simulink model "work"  (R2023a)
settings: Solver=FixedStepDiscrete  StartTime=1  StopTime=16  FixedStep=1  RelTol=1e-3
model workspace (MAT data in the model file):
  efwed = 0
undefined symbols (not defined in the file or in its folder): kfailsoftroll, mode
libraries: simulink x7
settings Model: DataDictionary=data.sldd  Creator=23208  LastModifiedBy=23208
settings DataIOCC: ExternalInput=[cycle, leftAdverseYaw,rightAdverseYaw,joystickCmd,expectationrollrate,OffPressed,expectationleftwarning,expectationrightwarning,expectationmode]  LoadExternalInput=on

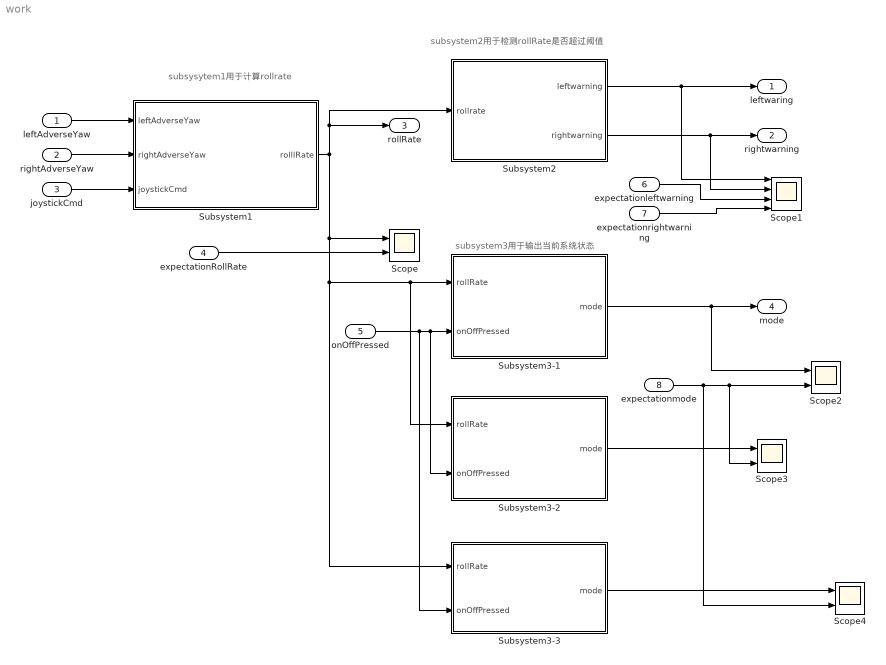
== system work ==
  note: subsystem2用于检测rollRate是否超过阈值
  note: subsysytem1用于计算rollrate
  note: subsystem3用于输出当前系统状态
  leftAdverseYaw : Inport  OutDataTypeStr=double
  rightAdverseYaw : Inport  Port=2  OutDataTypeStr=double
  joystickCmd : Inport  Port=3  OutDataTypeStr=double
  expectationRollRate : Inport  Port=4
  onOffPressed : Inport  Port=5
  expectationleftwarning : Inport  Port=6  OutDataTypeStr=double
  expectationrightwarning : Inport  Port=7  OutDataTypeStr=double
  expectationmode : Inport  Port=8
  Scope{,2..4} (4 alike) : Scope  NumInputPorts=2
  Scope1 : Scope  NumInputPorts=4
  Subsystem1 : Subsystem
  Subsystem2 : Subsystem
  Subsystem3-1 : Subsystem
  Subsystem3-2 : Subsystem
  Subsystem3-3 : Subsystem
  leftwaring : Outport  OutDataTypeStr=boolean
  rightwarning : Outport  Port=2  OutDataTypeStr=boolean
  rollRate : Outport  Port=3
  mode : Outport  Port=4
  wires:
  leftAdverseYaw/1 -> Subsystem1/1(leftAdverseYaw)
  rightAdverseYaw/1 -> Subsystem1/2(rightAdverseYaw)
  Subsystem1/1(rolllRate) -> Subsystem3-3/1(rollRate), Subsystem3-2/1(rollRate), Subsystem3-1/1(rollRate), Scope/1, rollRate/1, Subsystem2/1(rollrate)
  Subsystem2/1(leftwarning) -> Scope1/1, leftwaring/1
  Subsystem2/2(rightwarning) -> Scope1/2, rightwarning/1
  joystickCmd/1 -> Subsystem1/3(joystickCmd)
  onOffPressed/1 -> Subsystem3-3/2(onOffPressed), Subsystem3-2/2(onOffPressed), Subsystem3-1/2(onOffPressed)
  Subsystem3-1/1(mode) -> Scope2/1, mode/1
  expectationRollRate/1 -> Scope/2
  expectationleftwarning/1 -> Scope1/3
  expectationrightwarning/1 -> Scope1/4
  expectationmode/1 -> Scope4/2, Scope3/2, Scope2/2
  Subsystem3-2/1(mode) -> Scope3/1
  Subsystem3-3/1(mode) -> Scope4/1

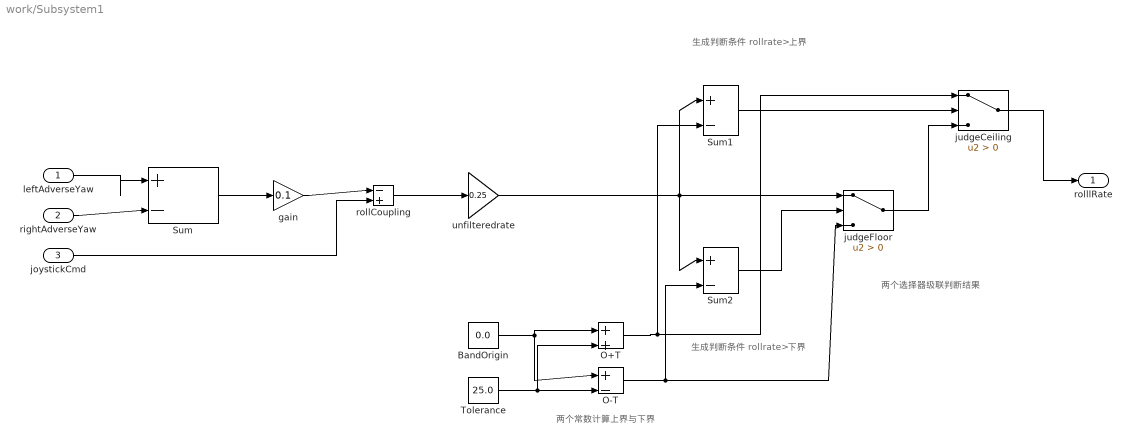
== system work/Subsystem1 ==
  note: 两个常数计算上界与下界
  note: 生成判断条件
      | rollrate>上界
  note: 生成判断条件
      | rollrate>下界
  note: 两个选择器级联判断结果
  leftAdverseYaw : Inport  OutDataTypeStr=double
  rightAdverseYaw : Inport  Port=2  OutDataTypeStr=double
  joystickCmd : Inport  Port=3  OutDataTypeStr=double
  BandOrigin : Constant  Value=0.0
  O+T : Sum  Inputs=|++
  O-T : Sum  Inputs=|+-
  Sum : Sum  Inputs=|+-
  Sum1 : Sum  Inputs=|+-
  Sum2 : Sum  Inputs=|+-
  Tolerance : Constant  Value=25.0
  gain : Gain  Gain=0.1
  judgeCeiling : Switch  Criteria=u2 > Threshold  SaturateOnIntegerOverflow=off  InputSameDT=off
  judgeFloor : Switch  Criteria=u2 > Threshold  SaturateOnIntegerOverflow=off  InputSameDT=off
  rollCoupling : Sum  Inputs=|-+
  unfilteredrate : Gain  Gain=0.25
  rolllRate : Outport  OutDataTypeStr=double
  wires:
  gain/1 -> rollCoupling/1
  BandOrigin/1 -> O-T/1, O+T/1
  Sum/1 -> gain/1
  Tolerance/1 -> O-T/2, O+T/2
  rightAdverseYaw/1 -> Sum/2
  judgeFloor/1 -> judgeCeiling/3
  leftAdverseYaw/1 -> Sum/1
  joystickCmd/1 -> rollCoupling/2
  rollCoupling/1 -> unfilteredrate/1
  unfilteredrate/1 -> judgeFloor/1, Sum1/1, Sum2/1
  O-T/1 -> Sum2/2, judgeFloor/3
  Sum2/1 -> judgeFloor/2
  Sum1/1 -> judgeCeiling/2
  O+T/1 -> judgeCeiling/1, Sum1/2
  judgeCeiling/1 -> rolllRate/1

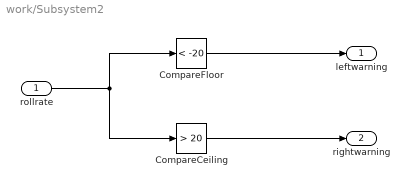
== system work/Subsystem2 ==
  rollrate : Inport
  CompareCeiling : simulink/Logic and Bit Operations/Compare To Constant  relop=>  const=20  OutDataTypeStr=boolean
  "CompareFloor " : simulink/Logic and Bit Operations/Compare To Constant  relop=<  const=-20  OutDataTypeStr=boolean
  leftwarning : Outport
  rightwarning : Outport  Port=2
  wires:
  CompareCeiling/1 -> rightwarning/1
  "CompareFloor "/1 -> leftwarning/1
  rollrate/1 -> "CompareFloor "/1, CompareCeiling/1

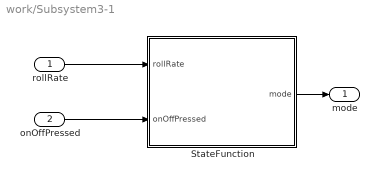
== system work/Subsystem3-1 ==
  rollRate : Inport
  onOffPressed : Inport  Port=2
  StateFunction : MATLAB Function  TreatAsAtomicUnit=on
  mode : Outport
  wires:
  rollRate/1 -> StateFunction/1(rollRate)
  onOffPressed/1 -> StateFunction/2(onOffPressed)
  StateFunction/1(mode) -> mode/1

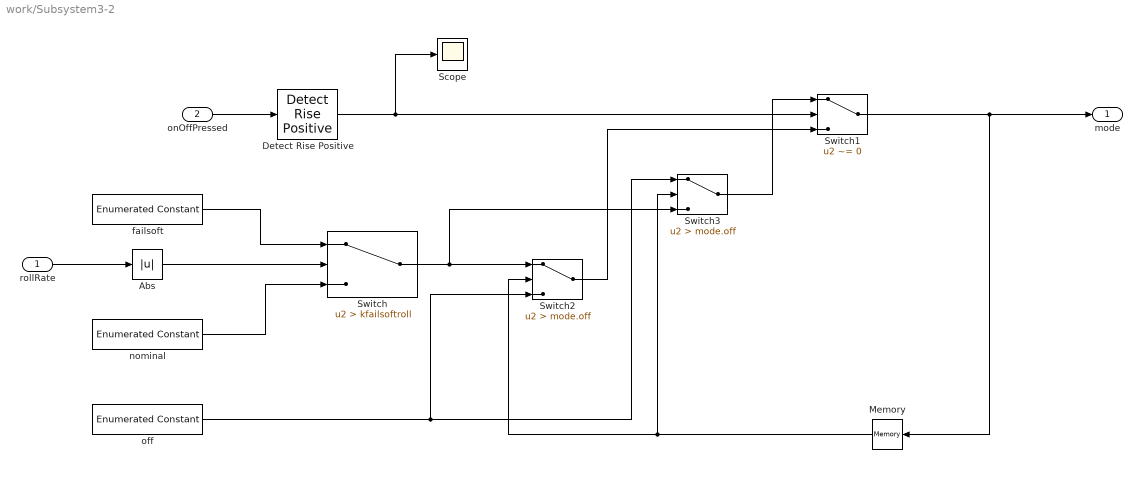
== system work/Subsystem3-2 ==
  rollRate : Inport
  onOffPressed : Inport  Port=2
  Abs : Abs  SaturateOnIntegerOverflow=off
  Detect Rise Positive : simulink/Logic and Bit Operations/Detect Rise Positive  vinit=1  OutDataTypeStr=boolean
  Memory : Memory  InitialCondition=mode.off
  Scope : Scope
  Switch : Switch  Criteria=u2 > Threshold  Threshold=kfailsoftroll  SaturateOnIntegerOverflow=off  InputSameDT=off
  Switch1 : Switch  Criteria=u2 ~= 0  SaturateOnIntegerOverflow=off  InputSameDT=off
  Switch2 : Switch  Criteria=u2 > Threshold  Threshold=mode.off  SaturateOnIntegerOverflow=off  InputSameDT=off
  Switch3 : Switch  Criteria=u2 > Threshold  Threshold=mode.off  SaturateOnIntegerOverflow=off  InputSameDT=off
  failsoft : simulink/Sources/Enumerated Constant  OutDataTypeStr=Enum: mode  Value=mode.failsoft  SampleTime=inf
  nominal : simulink/Sources/Enumerated Constant  OutDataTypeStr=Enum: mode  Value=mode.nominal  SampleTime=inf
  off : simulink/Sources/Enumerated Constant  OutDataTypeStr=Enum: mode  Value=mode.off  SampleTime=inf
  mode : Outport
  wires:
  rollRate/1 -> Abs/1
  Abs/1 -> Switch/2
  onOffPressed/1 -> Detect Rise Positive/1
  Detect Rise Positive/1 -> Scope/1, Switch1/2
  nominal/1 -> Switch/3
  failsoft/1 -> Switch/1
  Memory/1 -> Switch3/2, Switch2/2
  Switch/1 -> Switch3/3, Switch2/1
  Switch1/1 -> Memory/1, mode/1
  Switch2/1 -> Switch1/3
  off/1 -> Switch2/3, Switch3/1
  Switch3/1 -> Switch1/1

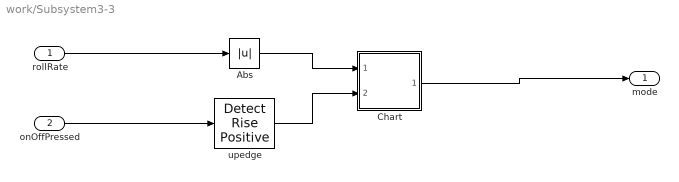
== system work/Subsystem3-3 ==
  rollRate : Inport
  onOffPressed : Inport  Port=2
  Abs : Abs  SaturateOnIntegerOverflow=off
  Chart : Stateflow chart  TreatAsAtomicUnit=on
  upedge : simulink/Logic and Bit Operations/Detect Rise Positive  vinit=1  OutDataTypeStr=boolean
  mode : Outport
  wires:
  upedge/1 -> Chart/2(upedge)
  onOffPressed/1 -> upedge/1
  rollRate/1 -> Abs/1
  Abs/1 -> Chart/1(rollRate)
  Chart/1(mode) -> mode/1

== matlab function work/Subsystem3-1/StateFunction ==
  data: rollRate input; mode output; onOffPressed input
function mode = calcSystemMode(rollRate, onOffPressed)
    % 定义枚举值
    OFF = 0;
    NOMINAL = 1;
    FAILSOFT = 2;
    persistent preonOffPressed;
    persistent prevMode;
    persistent systemState;
    %定义阈值常量
    kFailSoftRoll = 20;
    %定义上升沿改变系统状态


    if isempty(prevMode)  % 第一个周期初始化为OFF状态
        prevMode = OFF;
        preonOffPressed = onOffPressed;
         mode = OFF;
        systemState = false;
        return;
    end
    if(preonOffPressed == 0 &&  onOffPressed == 1)
        systemState = ~systemState;
    end
    mode = prevMode;
    %OFF状态判断
    if((prevMode == NOMINAL ||prevMode ==FAILSOFT) &&~systemState)
        mode = OFF;
    end

    %NOMINAL状态判断
    if(prevMode == OFF && systemState && abs(rollRate)<=kFailSoftRoll)
        mode = NOMINAL;
    end
    if(prevMode == FAILSOFT && abs(rollRate)<=kFailSoftRoll)
        mode = NOMINAL;
    end

    %FAILSOFT状态判断
    if(prevMode == OFF && systemState && abs(rollRate)>kFailSoftRoll)
        mode = FAILSOFT;
    end

    if(prevMode == NOMINAL&& abs(rollRate)>kFailSoftRoll)
        mode = FAILSOFT;
    end
    preonOffPressed = onOffPressed;
    prevMode = mode;
end

== stateflow chart work/Subsystem3-3/Chart ==
  state failsoft
    mode = 2
  state off
    mode = 0
  state nominal
    mode = 1
  failsoft -> off [order 2] : [upedge]
  (default) -> off
  off -> failsoft [order 1] : [upedge&&rollRate>20]
  failsoft -> nominal [order 1] : [rollRate<=20]
  nominal -> failsoft [order 1] : [rollRate>20]
  nominal -> off [order 2] : [upedge]
  off -> nominal [order 2] : [upedge&&rollRate<=20]
  data: rollRate input; upedge input; mode output
